simulink model "Tractive_System_model"  (R2025b)
settings: Solver=ode15s  StartTime=0  StopTime=85  MaxStep=1e-5  MinStep=1e-8  RelTol=1e-3  AbsTol=1e-6
undefined symbols (not defined in the file): FL, FR, RL, RR
libraries: batteryecm_lib x280, fl_lib x56, nesl_utility x37, ee_lib x9, sdl_lib x9, simulink x1, slpidlib x1, autolibshared x1, eePmsmFieldOrientedControl x1, eePmsmFwController x1
(part 1 of 23)
settings Model: PacingRate=0.002200  Creator=muizz  LastModifiedBy=muizz
settings SolverCC: AutoScaleAbsTol=off  InitialStep=1e-6  MaxConsecutiveMinStep=10000  ZeroCrossAlgorithm=Adaptive
settings DebuggingCC: AlgebraicLoopMsg=none  IgnoredZcDiagnostic=none

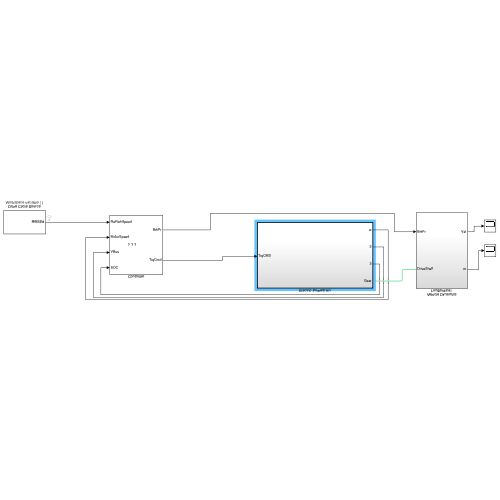
[thumbnail: Simulink's stored preview of the top-level diagram]
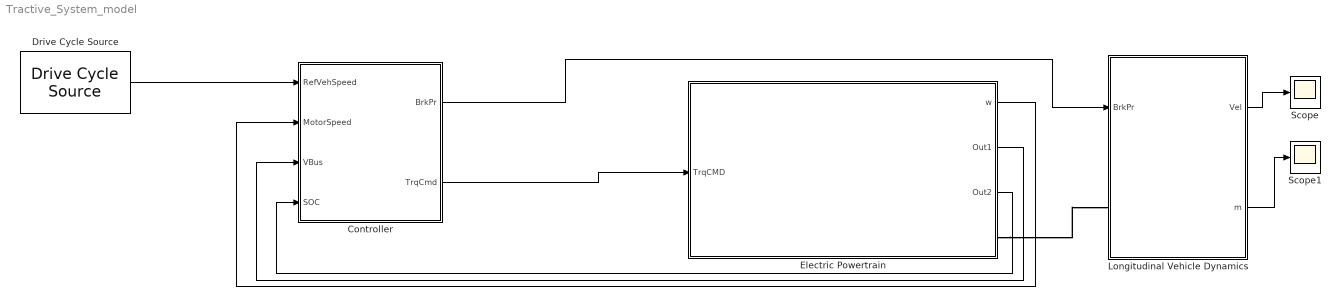
== system Tractive_System_model ==
  Controller : Subsystem
      mask Display: image('Images/brakeThrottle.png'); % Use "Edit Image" on toolstrip to change.
  Drive Cycle Source : autolibshared/Drive Cycle Source  cycleVar=Workspace variable  wsVar=fsdCycle  fileVar=cycleFTP75.mat  tfinal=""  cycleRepeat=on  outAccPort=off  outGearPort=off  gearList=No gear data  t_wot1=5  xdot_woto=0  xdot_wot1=30  t_wot2=20  xdot_wot2=0  t_wotend=30  srcUnit=m/s  outUnit=km/h  srcAccUnit=m/s/s  outAccUnit=m/s^2  dt=0  aMode=1  faultOption=off  velBnd=2  velBndUnit=mph  inUnit=m/s  timeBnd=1  failOption=off  stopSim=off  maxFaultCnt=10  maxFaultTime=2  maxTotFaultTime=15  traceOption=off  dtTrace=1  traceWindow=10  lastDCname=Custom Data Set  lastOutUnit=mph  lastDT=0  lastTB=1  lastSB=2  forceCalcBound=off
  Electric Powertrain : Subsystem  TreatAsAtomicUnit=on
  Longitudinal Vehicle Dynamics : Subsystem
  Scope : Scope
      settings: ActiveDisplayYMinimum=-1.2426886947971694  ActiveDisplayYMaximum=4.3208277664924974  DataLoggingVariableName=ScopeData5
  Scope1 : Scope
      settings: ActiveDisplayYMinimum=-1.4911055612240759E-16  ActiveDisplayYMaximum=1.5005598990985852E-16  DataLoggingVariableName=ScopeData6
  wires:
  Controller/2(TrqCmd) -> Electric Powertrain/1(TrqCMD)
  Electric Powertrain/1(w) -> Controller/2(MotorSpeed)
  Controller/1(BrkPr) -> Longitudinal Vehicle Dynamics/1(BrkPr)
  Drive Cycle Source/1 -> Controller/1(RefVehSpeed)
  Longitudinal Vehicle Dynamics/2(m) -> Scope1/1
  Longitudinal Vehicle Dynamics/1(Vel) -> Scope/1
  Electric Powertrain/2(Out1) -> Controller/3(VBus)
  Electric Powertrain/3(Out2) -> Controller/4(SOC)
  connections:
  Electric Powertrain/RConn1 -- Longitudinal Vehicle Dynamics/LConn1

== system Tractive_System_model/Controller ==
  RefVehSpeed : Inport
  MotorSpeed : Inport  Port=2
  VBus : Inport  Port=3
  SOC : Inport  Port=4
  Control : Subsystem
  Motor Speed Reference : Subsystem
  BrkPr : Outport
  TrqCmd : Outport  Port=2
  tag scope: Ref=global
  wires:
  RefVehSpeed/1 -> [Ref], Motor Speed Reference/1(VehSpd)
  MotorSpeed/1 -> Control/1(In1)
  Motor Speed Reference/1(MotorSpdRef) -> Control/2(Motor Speed Ref)  "Motor Speed Ref"
  VBus/1 -> Control/3(VBus)
  SOC/1 -> Control/4(SOC)
  Control/1(Pressure) -> BrkPr/1
  Control/2(MotCmdTrq) -> TrqCmd/1

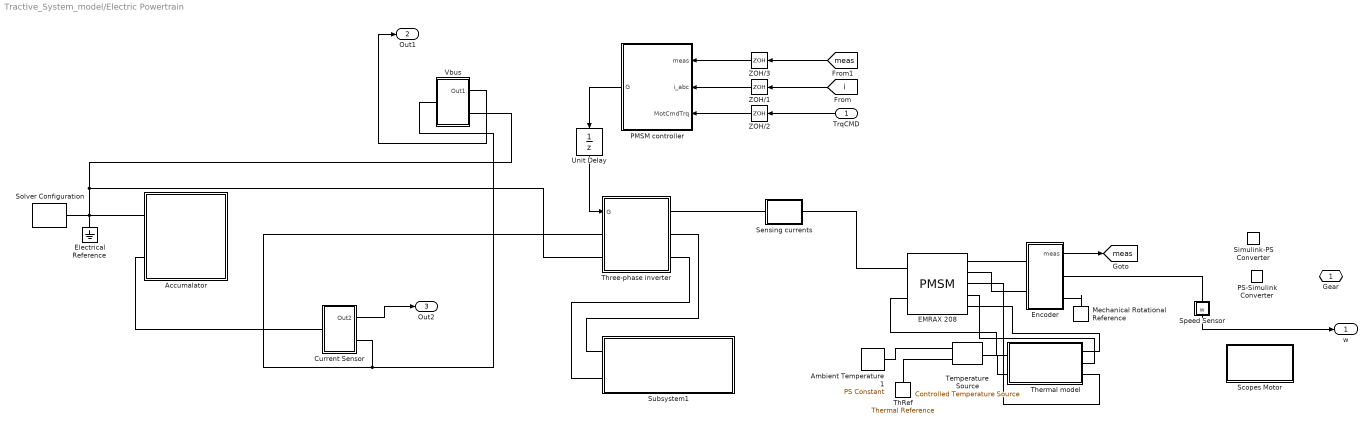
== system Tractive_System_model/Electric Powertrain ==
  TrqCMD : Inport
  Accumalator : Subsystem
  Ambient Temperature1 : fl_lib/Physical Signals/Sources/PS Constant  constant=300.15 K
  Current Sensor : Subsystem
  EMRAX 208 : ee_lib/Electromechanical/Permanent Magnet/PMSM  port_option=ee.enum.threePhasePort.composite  winding_type=ee.enum.electromech.statorconfiguration.wye  machine_param=ee.enum.pmsm.parameterization.constant  nPolePairs=10  pmflux_param=ee.enum.pmflux.fluxlinkage  pm_flux_linkage=0.23 Wb  torque_constant=0.916923438250803 % Datasheet derived N*m/A  back_emf_constant=0.916923438250803 % Datasheet derived V/(rad/s)  stator_param=ee.enum.statorparam.LdLqL0  Ld=0.138 mH  Lq=0.138 mH  idVec=[-200, 0, 200] A  iqVec=[-200, 0, 200] A  LdMatrix=0.0002 * ones(3, 3) H  LqMatrix=0.0002 * ones(3, 3) H  PmMatrix=0.1 * ones(3, 3) Wb  ktMatrix=0.18 * ones(3, 3) N*m/A  keMatrix=0.18 * ones(3, 3) V*s/rad  L0=0.00016 H  Ls=0.0002 H  Lm=-0.00002 H  Ms=0.00002 H  Rs=12 mOhm  zero_sequence=ee.enum.park.zerosequence.exclude  axes_param=ee.enum.rotorangle.daxis  loss_param=ee.enum.ironloss.none  losses_oc=[0, 0, 0] W  losses_sc=[0, 0, 0] W  f_losses=60 Hz  Isc_losses=95 A  J=256 kg*cm^2  lam=0 N*m*s/rad  i_d_specify=off  i_d_priority=None  i_d=0 A  i_d_nominal_specify=off  i_d_nominal_value=1  i_d_nominal_unit=A  i_q_specify=off  i_q_priority=None  i_q=0 A  i_q_nominal_specify=off  i_q_nominal_value=1  i_q_nominal_unit=A  torque_specify=off  torque_priority=High  torque=80 N*m  torque_nominal_specify=on  torque_nominal_value=80  torque_nominal_unit=N*m  angular_velocity_specify=off  angular_velocity_priority=High  angular_velocity=0 rpm  angular_velocity_nominal_specify=off  angular_velocity_nominal_value=1  angular_velocity_nominal_unit=rpm  angular_position_specify=off  angular_position_priority=High  angular_position=0 deg  angular_position_nominal_specify=off  angular_position_nominal_value=1  angular_position_nominal_unit=deg  alpha=3.93e-3 1/K  alpha_flux=-0.001 1/K  Tmeas=298.15 K  stator_thermal_mass=423.5 J/K  rotor_thermal_mass=2714 J/K  Rm_percent_rotor=90  Rd_percent_rotor=30  temperatureA_specify=off  temperatureA_priority=High  temperatureA=25 degC  temperatureA_nominal_specify=off  temperatureA_nominal_value=1  temperatureA_nominal_unit=degC  temperatureB_specify=off  temperatureB_priority=High  temperatureB=25 degC  temperatureB_nominal_specify=off  temperatureB_nominal_value=1  temperatureB_nominal_unit=degC  temperatureC_specify=off  temperatureC_priority=High  temperatureC=25 degC  temperatureC_nominal_specify=off  temperatureC_nominal_value=1  temperatureC_nominal_unit=degC  temperatureR_specify=off  temperatureR_priority=High  temperatureR=25 degC  temperatureR_nominal_specify=off  temperatureR_nominal_value=1  temperatureR_nominal_unit=degC
      settings: InternalSimscapePortConfiguration="{\"Bottom\":[],\"Left\":[{\"id\":\"N\",\"label\":\"~\",\"type\":\"foundation.electrical.three_phase\"},{\"id\":\"HR\",\"label\":\"HR\",\"type\":\"foundation.thermal.thermal\"}],\"Right\":[{\"id\":\"R\",\"label\":\"R\",\"type\":\"foundation.mechanical.rotational.rotational\"},{\"id\":\"C\",\"label\":\"C\",\"type\":\"foundation.mechanical.rotational.rotational\"},{\"id\":\"HA\",\"label\":\"HA\",\"type\":\"foundation.thermal.thermal\"},{\"id\":\"HB\",\"label\":\"HB\",\"type\":\"foundation.thermal.thermal\"},{\"id\":\"HC\",\"label\":\"HC\",\"type\":\"foundation.thermal.thermal\"}],\"Top\":[]}"
  Electrical Reference : fl_lib/Electrical/Electrical Elements/Electrical Reference
  Encoder : Subsystem
  Mechanical Rotational Reference : fl_lib/Mechanical/Rotational Elements/Mechanical Rotational Reference
  PMSM controller : Subsystem
  PS-Simulink Converter : nesl_utility/PS-Simulink Converter  PhysicalDomain=network_engine_domain  SubClassName=ps_output  LeftPortType=input  RightPortType=output  PseudoPeriodic=off  Frequencies=[]  VectorFormat=inherit  Unit=inherit  AffineConversion=off
  Scopes Motor : Subsystem
  Sensing currents : Subsystem
      mask Display: disp('i')
  Simulink-PS Converter : nesl_utility/Simulink-PS Converter  PhysicalDomain=network_engine_domain  SubClassName=ps_input  LeftPortType=input  RightPortType=output  PseudoPeriodic=off  Frequencies=[]  NoiseDistribution=none  NoiseParameters=[]  Unit=1  AffineConversion=off  FilteringAndDerivatives=provide  SimscapeFilterOrder=1  InputFilterTimeConstant=0.001  UdotUserProvided=0
  Solver Configuration : nesl_utility/Solver Configuration  PhysicalDomain=network_engine_domain  SubClassName=solver  LeftPortType=input  RightPortType=generic  Tones=[]  Harmonics=[]  SimulateNoise=off  Profile=off  UseLocalSampling=off  EnableSwitchedLinearOptims=on  FrequencyDomain=off  UseCCode=off  RelTol=0.001  AbsTol=0.001  MinStep=1e-09  ToWorkspace=off  RevertToSquareIcSolve=off  NumHomotopyIterations=100  PhasorMode=off  PhasorModeNumHarmonics=1  ConsistencySolver=NEWTON_XTOL_AFTER_FTOL  IndexReductionMethod=DerivativeReplacement  DoDC=off  ResidualTolerance=1e-09  ConsistencyTolSource=GLOBAL  ConsistencyAbsTol=0.001  ConsistencyRelTol=0.001  ConsistencyTolFactor=1e-4  UseLocalSolver=off  LocalSolverChoice=NE_BACKWARD_EULER_ADVANCER  ResolveIndetEquations=on  FunctionEvalNumThread=1  LocalSolverSampleTime=1e-04  DoFixedCost=off  MaxNonlinIter=3  MaxModeIter=2  ComputeImpulses=off  ImpulseIterations=2  LinearAlgebra=auto  LinearAlgebraNumThread=0  EquationFormulation=NE_TIME_EF  DelaysMemoryBudget=1024  AutomaticFiltering=on  FilteringTimeConstant=0.001  PartitionStorageMethod=AS_NEEDED  PartitionMemoryBudget=1024  PartitionMethod=ROBUST  MultibodyUseLocalSolver=off  MultibodyLocalSolverChoice=ODE1  MultibodyLocalSolverSampleTime=0.005
  Speed Sensor : Subsystem
      mask Display: disp('w')
  Subsystem1 : Subsystem
  Temperature Source : fl_lib/Thermal/Thermal Sources/Controlled Temperature Source
  ThRef : fl_lib/Thermal/Thermal Elements/Thermal Reference
  Thermal model : Subsystem  Tag=PublishSubsystem
  Three-phase inverter : Subsystem
  Unit Delay : UnitDelay  SampleTime=-1  HasFrameUpgradeWarning=on
  Vbus : Subsystem
  ZOH/1 : ZeroOrderHold  SampleTime=2e-05
  ZOH/2 : ZeroOrderHold  SampleTime=2e-05
  ZOH/3 : ZeroOrderHold  SampleTime=2e-05
  Gear : PMIOPort  Side=Right
  w : Outport
  Out1 : Outport  Port=2
  Out2 : Outport  Port=3
  tag scope: meas=global
  wires:
  Unit Delay/1 -> Three-phase inverter/1(G)
  [meas] -> ZOH/3/1
  PMSM controller/1(G) -> Unit Delay/1
  Speed Sensor/1(w) -> w/1
  Encoder/1(meas) -> [meas]
  [i] -> ZOH/1/1
  ZOH/2/1 -> PMSM controller/3(MotCmdTrq)
  ZOH/1/1 -> PMSM controller/2(i_abc)
  ZOH/3/1 -> PMSM controller/1(meas)
  TrqCMD/1 -> ZOH/2/1
  Current Sensor/1(Out2) -> Out2/1
  Vbus/1(Out1) -> Out1/1
  connections:
  EMRAX 208/RConn2 -- Encoder/LConn2
  Thermal model/RConn1 -- EMRAX 208/RConn5
  Temperature Source/LConn1 -- Thermal model/LConn2
  Sensing currents/LConn1 -- Three-phase inverter/RConn1
  ThRef/LConn1 -- Temperature Source/RConn2
  Temperature Source/RConn1 -- Ambient Temperature1/RConn1
  EMRAX 208/RConn4 -- Thermal model/RConn2
  Speed Sensor/LConn1 -- Encoder/RConn1
  Sensing currents/RConn1 -- EMRAX 208/LConn1
  Three-phase inverter/LConn2 -- Vbus/RConn1 -- Solver Configuration/RConn1 -- Electrical Reference/LConn1 -- Accumalator/LConn1
  Thermal model/RConn3 -- EMRAX 208/RConn3
  EMRAX 208/RConn1 -- Encoder/LConn1
  Mechanical Rotational Reference/LConn1 -- Encoder/RConn2
  Thermal model/LConn1 -- EMRAX 208/LConn2
  Three-phase inverter/RConn2 -- Subsystem1/LConn1
  Three-phase inverter/RConn3 -- Subsystem1/LConn2
  Current Sensor/LConn1 -- Accumalator/LConn2
  Current Sensor/RConn1 -- Vbus/LConn1 -- Three-phase inverter/LConn1

== system Tractive_System_model/Longitudinal Vehicle Dynamics ==
  BrkPr : Inport
  Brakes : Subsystem
  Bus Selector2 : BusSelector  OutputSignals=RoadGrade,Wind
  Chassis and Tires : Subsystem
  Env : Subsystem
  PS Gain1 : fl_lib/Physical Signals/Functions/PS Gain  gain=1
  Sensor Subsystem : Subsystem
  Simulink-PS Converter : nesl_utility/Simulink-PS Converter  PhysicalDomain=network_engine_domain  SubClassName=ps_input  LeftPortType=input  RightPortType=output  PseudoPeriodic=off  Frequencies=[]  NoiseDistribution=none  NoiseParameters=[]  Unit=1  AffineConversion=off  FilteringAndDerivatives=provide  SimscapeFilterOrder=1  InputFilterTimeConstant=0.001  UdotUserProvided=0
  Simulink-PS Converter2 : nesl_utility/Simulink-PS Converter  PhysicalDomain=network_engine_domain  SubClassName=ps_input  LeftPortType=input  RightPortType=output  PseudoPeriodic=off  Frequencies=[]  NoiseDistribution=none  NoiseParameters=[]  Unit=rad  AffineConversion=off  FilteringAndDerivatives=provide  SimscapeFilterOrder=1  InputFilterTimeConstant=0.001  UdotUserProvided=0
  Simulink-PS Converter3 : nesl_utility/Simulink-PS Converter  PhysicalDomain=network_engine_domain  SubClassName=ps_input  LeftPortType=input  RightPortType=output  PseudoPeriodic=off  Frequencies=[]  NoiseDistribution=none  NoiseParameters=[]  Unit=N/m^2  AffineConversion=off  FilteringAndDerivatives=provide  SimscapeFilterOrder=1  InputFilterTimeConstant=0.001  UdotUserProvided=0
  Simulink-PS Converter4 : nesl_utility/Simulink-PS Converter  PhysicalDomain=network_engine_domain  SubClassName=ps_input  LeftPortType=input  RightPortType=output  PseudoPeriodic=off  Frequencies=[]  NoiseDistribution=none  NoiseParameters=[]  Unit=m/s  AffineConversion=off  FilteringAndDerivatives=provide  SimscapeFilterOrder=1  InputFilterTimeConstant=0.001  UdotUserProvided=0
  DriveShaft : PMIOPort  Side=Left
  Vel : Outport
  Out Bus Element : Outport  Port=2  PortName=m  Element=Brakes
  Out Bus Element1 : Outport  Port=2  PortName=m  Element=Chassis
  wires:
  BrkPr/1 -> Simulink-PS Converter3/1
  Env/1(Env) -> Bus Selector2/1
  Brakes/1(m) -> Out Bus Element/1
  Bus Selector2/2 -> Simulink-PS Converter4/1  "<Wind>"
  Bus Selector2/1 -> Simulink-PS Converter2/1  "<RoadGrade>"
  Chassis and Tires/1(m) -> Out Bus Element1/1
  Sensor Subsystem/1(kph) -> Vel/1, Env/1(m)
  connections:
  PS Gain1/LConn1 -- Brakes/LConn1 -- Simulink-PS Converter3/RConn1
  Chassis and Tires/RConn2 -- Simulink-PS Converter4/RConn1
  PS Gain1/RConn1 -- Brakes/LConn2
  Chassis and Tires/LConn2 -- DriveShaft/RConn1
  Chassis and Tires/LConn1 -- Brakes/RConn1
  Chassis and Tires/RConn1 -- Simulink-PS Converter2/RConn1
  Chassis and Tires/RConn3 -- Sensor Subsystem/LConn1

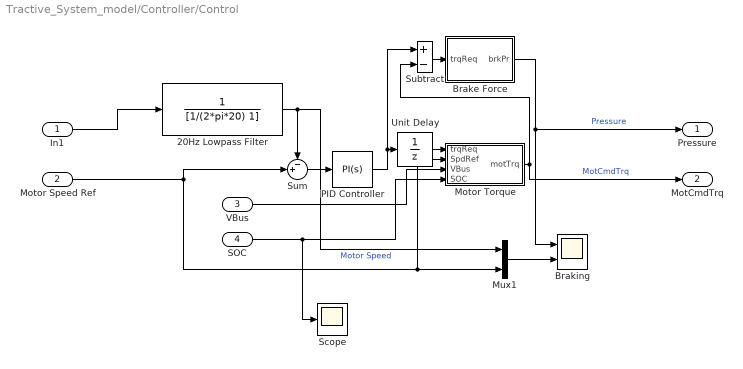
== system Tractive_System_model/Controller/Control ==
  In1 : Inport
  Motor Speed Ref : Inport  Port=2
  VBus : Inport  Port=3
  SOC : Inport  Port=4
  20Hz Lowpass Filter : TransferFcn  Denominator=[1/(2*pi*20) 1]
  Brake Force : Subsystem
  Braking : Scope  NumInputPorts=2
      settings: ActiveDisplayYMinimum=-6.26637814618E+6  ActiveDisplayYMaximum=5.639740331562E+7
  Motor Torque : Subsystem
  Mux1 : Mux  Inputs=2
  PID Controller : slpidlib/PID Controller  Controller=PI  Form=Parallel  TimeDomain=Continuous-time  UseExternalTs=off  SampleTime=-1  IntegratorMethod=Forward Euler  FilterMethod=Forward Euler  ControllerParametersSource=internal  P=0.5  I=1e-03  UseKiTs=off  D=0  UseExternalDerivativeSource=off  N=100  UseFilter=on  TunerSelectOption=Transfer Function Based (PID Tuner App)  InitialConditionSource=internal  InitialConditionForIntegrator=0  InitialConditionForFilter=0  DifferentiatorICPrevScaledInput=0  ExternalReset=none  TrackingMode=off  Kt=1  LimitOutput=off  SatLimitsSource=internal  UpperSaturationLimit=inf  LowerSaturationLimit=-inf  LinearizeAsGain=on  AntiWindupMode=none  Kb=1  LimitIntegrator=off  UpperIntegratorSaturationLimit=inf  LowerIntegratorSaturationLimit=-inf  POutMin=[]  POutMax=[]  IOutMin=[]  IOutMax=[]  DOutMin=[]  DOutMax=[]  NOutMin=[]  NOutMax=[]  SumOutMin=[]  SumOutMax=[]  SaturationOutMin=[]  SaturationOutMax=[]  PParamMin=[]  PParamMax=[]  IParamMin=[]  IParamMax=[]  DParamMin=[]  DParamMax=[]  NParamMin=[]  NParamMax=[]  KbParamMin=[]  KbParamMax=[]  KtParamMin=[]  KtParamMax=[]  KbOutMin=[]  KbOutMax=[]  KtOutMin=[]  KtOutMax=[]  IntegratorOutMin=[]  IntegratorOutMax=[]  FilterOutMin=[]  FilterOutMax=[]  SumI1OutMin=[]  SumI1OutMax=[]  SumI2OutMin=[]  SumI2OutMax=[]  SumI3OutMin=[]  SumI3OutMax=[]  SumI4OutMin=[]  SumI4OutMax=[]  SumDOutMin=[]  SumDOutMax=[]  DifferentiatorOutMin=[]  DifferentiatorOutMax=[]  FilterDiffOutCoefMin=[]  FilterDiffOutCoefMax=[]  ReciprocalOutMin=[]  ReciprocalOutMax=[]  SumDenOutMin=[]  SumDenOutMax=[]  SumNumOutMin=[]  SumNumOutMax=[]  DivideOutMin=[]  DivideOutMax=[]  UdiffTsProdOutMin=[]  UdiffTsProdOutMax=[]  NTsProdOutMin=[]  NTsProdOutMax=[]  UintegralTsProdOutMin=[]  UintegralTsProdOutMax=[]  UngainTsProdOutMin=[]  UngainTsProdOutMax=[]  ClampingZeroOutDataTypeStr=Inherit: Inherit via back propagation  ClampingZeroOutMin=[]  ClampingZeroOutMax=[]  FilterDenConstantOutDataTypeStr=Inherit: Inherit via back propagation  FilterDenConstantOutMin=[]  FilterDenConstantOutMax=[]  PCopyOutDataTypeStr=Inherit: Inherit via back propagation  PCopyOutMin=[]  PCopyOutMax=[]  NCopyOutDataTypeStr=Inherit: Inherit via back propagation  NCopyOutMin=[]  NCopyOutMax=[]  IntegratorContinuousStateAttributes=''  IntegratorStateMustResolveToSignalObject=off  IntegratorRTWStateStorageClass=Auto  FilterContinuousStateAttributes=''  FilterStateMustResolveToSignalObject=off  FilterRTWStateStorageClass=Auto  ParallelPVariant=InternalParameters  IdealPVariant=Disabled  IVariant=InternalParameters  DVariant=Disabled  IntegratorVariant=Continuous  SatVariant=Disabled  AWVariant=Passthrough  PCopyVariant=Disabled  TRVariant=Disabled  FdbkBlocksVariant=Forward  IdealPFdbkVariant=Disabled  SatFdbkVariant=Disabled  DerivativeFilterVariant=Disabled  NVariant=Disabled  NCopyVariant=Disabled_SignalSpec  FilterICVariant=Disabled  IntegratorICVariant=InternalICs  ExternalResetVariant=Disabled  TRSumVariant=Passthrough  SumFdbkVariant=Disabled  SumVariant=Sum_PI  TsampFilterVariant=InternalTs  TsampNgainVariant=Passthrough  TsampIntegralVariant=Disabled_SignalSpec  ExternalSaturationOutDataTypeStr=Inherit: Same as second input  DerivativeSourceVariant=Disabled  PreIntVariant=InternalPreInt
  Scope : Scope
      settings: DataLoggingVariableName=ScopeData7
  Subtract : Sum  Inputs=+-
  Sum : Sum  Inputs=-+|
  Unit Delay : UnitDelay  SampleTime=-1  HasFrameUpgradeWarning=on
  Pressure : Outport
  MotCmdTrq : Outport  Port=2
  wires:
  Sum/1 -> PID Controller/1
  Motor Torque/1(motTrq) -> MotCmdTrq/1, Subtract/2  "MotCmdTrq"
  20Hz Lowpass Filter/1 -> Sum/1, Mux1/1  "Motor Speed"
  Brake Force/1(brkPr) -> Pressure/1, Braking/1  "Pressure"
  Mux1/1 -> Braking/2
  Subtract/1 -> Brake Force/1(trqReq)
  Motor Speed Ref/1 -> Motor Torque/2(SpdRef), Mux1/2, Sum/2
  VBus/1 -> Motor Torque/3(VBus)
  SOC/1 -> Scope/1, Motor Torque/4(SOC)
  In1/1 -> 20Hz Lowpass Filter/1
  PID Controller/1 -> Subtract/1, Unit Delay/1
  Unit Delay/1 -> Motor Torque/1(trqReq)

== system Tractive_System_model/Controller/Motor Speed Reference ==
  note: Motor Reducer Output Shaft to Wheels
  VehSpd : Inport  Unit=km/hr
  Constant1 : Constant  Value=20.32
  Differential : Constant  Value=4.28
  Divide : Product  Inputs=*/
  Gain : Gain  Gain=2*pi
  Gain1 : Gain  Gain=1/100
  Product : Product
  Signal Specification : SignalSpecification  Unit=m/min
  Unit Conversion : UnitConversion
  MotorSpdRef : Outport  Unit=rpm  VectorParamsAs1DForOutWhenUnconnected=off
  wires:
  VehSpd/1 -> Unit Conversion/1
  Unit Conversion/1 -> Signal Specification/1
  Signal Specification/1 -> Divide/1
  Constant1/1 -> Gain1/1  "cm"
  Gain/1 -> Divide/2  "2*pi*R (m)"
  Divide/1 -> Product/1  "tireRpmRef"
  Product/1 -> MotorSpdRef/1  "motorRpmRef"
  Gain1/1 -> Gain/1  "m"
  Differential/1 -> Product/2

== system Tractive_System_model/Electric Powertrain/Accumalator ==
  Module  four : Subsystem
  Module Five1 : Subsystem
  Module One1 : Subsystem
  Module Three1 : Subsystem
  "Module Two " : Subsystem
  - : PMIOPort  Side=Left
  + : PMIOPort  Port=2  Side=Left
  connections:
  "Module Two "/LConn2 -- Module Three1/LConn1
  Module Three1/LConn2 -- Module  four/LConn1
  Module One1/LConn2 -- "Module Two "/LConn1
  Module  four/LConn2 -- Module Five1/LConn1
  Module Five1/LConn2 -- -/RConn1
  Module One1/LConn1 -- +/RConn1

== system Tractive_System_model/Electric Powertrain/Current Sensor ==
  Current Sensor : fl_lib/Electrical/Electrical Sensors/Current Sensor
  Current sensing : nesl_utility/PS-Simulink Converter  PhysicalDomain=network_engine_domain  SubClassName=ps_output  LeftPortType=input  RightPortType=output  PseudoPeriodic=off  Frequencies=[]  VectorFormat=inherit  Unit=inherit  AffineConversion=off
  Integrator : Integrator  InitialCondition=1
  Saturation : Saturate  UpperLimit=1  LowerLimit=0
  Scope1 : Scope
      settings: ActiveDisplayYMinimum=-20.563211553740629  ActiveDisplayYMaximum=64.19065525989943  DataLoggingVariableName=ScopeData4
  Conn1 : PMIOPort  Side=Left
  Conn2 : PMIOPort  Port=2  Side=Right
  Out2 : Outport
  wires:
  Saturation/1 -> Out2/1
  Current sensing/1 -> Integrator/1, Scope1/1
  Integrator/1 -> Saturation/1
  connections:
  Current Sensor/LConn1 -- Conn1/RConn1
  Current Sensor/RConn2 -- Conn2/RConn1
  Current Sensor/RConn1 -- Current sensing/LConn1

== system Tractive_System_model/Electric Powertrain/Encoder ==
  Ideal Rotational Motion Sensor : fl_lib/Mechanical/Mechanical Sensors/Ideal Rotational Motion Sensor  reference=foundation.enum.MeasurementReference.difference  acceleration_port=false  velocity_port=true  position_port=true  wrap_angle=simscape.enum.onoff.off  offset=0 deg
  Ideal Torque Sensor : fl_lib/Mechanical/Mechanical Sensors/Ideal Torque Sensor
  Mux : Mux  Inputs=2
  PS-Simulink Converter : nesl_utility/PS-Simulink Converter  PhysicalDomain=network_engine_domain  SubClassName=ps_output  LeftPortType=input  RightPortType=output  PseudoPeriodic=off  Frequencies=[]  VectorFormat=1-D array  Unit=rad/s  AffineConversion=off
  PS-Simulink Converter1 : nesl_utility/PS-Simulink Converter  PhysicalDomain=network_engine_domain  SubClassName=ps_output  LeftPortType=input  RightPortType=output  PseudoPeriodic=off  Frequencies=[]  VectorFormat=1-D array  Unit=rad  AffineConversion=off
  PS-Simulink Converter2 : nesl_utility/PS-Simulink Converter  PhysicalDomain=network_engine_domain  SubClassName=ps_output  LeftPortType=input  RightPortType=output  PseudoPeriodic=off  Frequencies=[]  VectorFormat=1-D array  Unit=N*m  AffineConversion=off
  1L : PMIOPort  Side=Left
  2L : PMIOPort  Port=2  Side=Left
  1R : PMIOPort  Port=3  Side=Right
  2R : PMIOPort  Port=4  Side=Right
  meas : Outport  VectorParamsAs1DForOutWhenUnconnected=off
  tag scope: trqMotor=global, wMotor=global
  wires:
  PS-Simulink Converter2/1 -> [trqMotor]
  Mux/1 -> meas/1
  PS-Simulink Converter1/1 -> Mux/2
  PS-Simulink Converter/1 -> [wMotor], Mux/1
  connections:
  Ideal Torque Sensor/RConn2 -- PS-Simulink Converter2/LConn1
  1L/RConn1 -- Ideal Torque Sensor/LConn1
  2R/RConn1 -- 2L/RConn1 -- Ideal Rotational Motion Sensor/RConn1
  Ideal Rotational Motion Sensor/LConn1 -- 1R/RConn1 -- Ideal Torque Sensor/RConn1
  Ideal Rotational Motion Sensor/RConn2 -- PS-Simulink Converter/LConn1
  Ideal Rotational Motion Sensor/RConn3 -- PS-Simulink Converter1/LConn1

== system Tractive_System_model/Electric Powertrain/PMSM controller ==
  meas : Inport
  i_abc : Inport  Port=2
  MotCmdTrq : Inport  Port=3
  Bus Selector : BusSelector  OutputSignals=iabc [A],Reference,TqRef [N*m],idq [A]
  Demux1 : Demux  Outputs=2
  PMSM Field-Oriented Control : eePmsmFieldOrientedControl/PMSM Field-Oriented Control  winding_type=Wye-wound  CtrlMode=Torque control  Vnom=572  Pmax=80000  Tmax=150  p=10  Vdc_on=30  Ts=1e-5  Tsc=1e-5  CtrlType=PI control  Kp_w=60  Ki_w=300*2  Kv_w=1  Kaw_w=1000  RefType=Zero d-axis control  rpmVec=[0, 3000]  TqVec=[-100, 0, 100]  VdcVec=[300, 350]  PWMMode=SPWM: sinusoidal PWM  ModFactor=1  idMatrix=zeros(2,3,2)  iqMatrix=zeros(2,3,2)  psim=0.0275  Ld=0.00024  Lq=0.00029  Rs=0.01  AxisAlignment=Q-axis  Kp_id=0.540  Ki_id=5.7  Kaw_id=1000  Kp_iq=0.540  Ki_iq=5.7  Kaw_iq=1000  AxisPrio=Q-axis  ActZC=off  ActFF=on  ParamTypeFF=Constant parameters  LdFF=0.0002  LqFF=0.0002  psimFF=0.0275  idVect=[-200, 0, 200]  iqVect=[-200, 0, 200]  LdMatrix=0.0002 * ones(3, 3)  LqMatrix=0.0002 * ones(3, 3)  psimMatrix=0.04 * ones(3, 3)  CPWMMode=SPWM: sinusoidal PWM  fsw=10000
  PMSM Field-Weakening Controller : eePmsmFwController/PMSM Field-Weakening Controller  Commented=on  Mth=1  Kfw=100  Kaw=10  Ts=-1
      settings: LibrarySourceBlock=|
      | ee_sl_lib/PMSM Control/PMSM Field-Weakening
      | Controller
  Vdc : Constant  Value=572  SampleTime=2e-05
  G : Outport  VectorParamsAs1DForOutWhenUnconnected=off
  tag scope: G=global, iMotor=global, idq=global, trqDemand=global, wDemand=global
  wires:
  PMSM Field-Oriented Control/1 -> G/1, [G]
  Vdc/1 -> PMSM Field-Oriented Control/5
  PMSM Field-Oriented Control/2 -> Bus Selector/1
  i_abc/1 -> PMSM Field-Oriented Control/2
  meas/1 -> Demux1/1
  Demux1/1 -> PMSM Field-Oriented Control/3
  Demux1/2 -> PMSM Field-Oriented Control/4
  Bus Selector/1 -> [iMotor]  "<iabc [A]>"
  Bus Selector/2 -> [wDemand]  "<Reference>"
  Bus Selector/3 -> [trqDemand]  "<TqRef [N*m]>"
  Bus Selector/4 -> [idq]  "<idq [A]>"
  MotCmdTrq/1 -> PMSM Field-Oriented Control/1

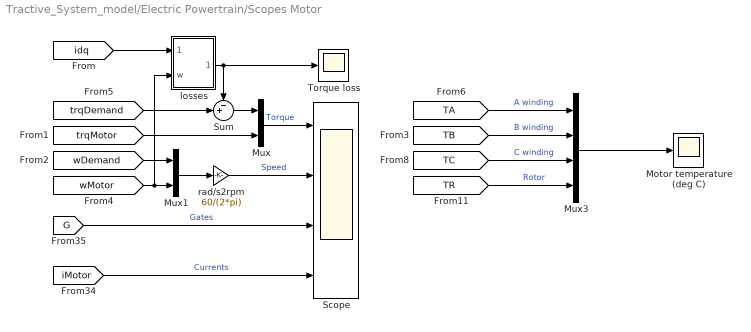
== system Tractive_System_model/Electric Powertrain/Scopes Motor ==
  Motor temperature (deg C) : Scope
      settings: Title=Motor temperature (deg C)  ActiveDisplayYMinimum=13.563074138954487  ActiveDisplayYMaximum=33.98024222270584  DataLoggingMaxPoints=500000  DataLoggingDecimation=10
  Mux : Mux  Inputs=2
  Mux1 : Mux  Inputs=2
  Mux3 : Mux
  Scope : Scope  NumInputPorts=4
      settings: Title=Demanded and achieved torques  ActiveDisplayYMinimum=-8.8227194148565182  ActiveDisplayYMaximum=43.531185116331216
  Sum : Sum  Inputs=-+|
  Torque loss : Scope
      settings: ActiveDisplayYMinimum=-15.776290162311993  ActiveDisplayYMaximum=9.8949447297595938
  losses : Subsystem
  rad/s2rpm : Gain  Gain=60/(2*pi)
  wires:
  [TC] -> Mux3/3  "C winding"
  [TR] -> Mux3/4  "Rotor"
  [TB] -> Mux3/2  "B winding"
  [TA] -> Mux3/1  "A winding"
  Mux3/1 -> Motor temperature (deg C)/1
  rad/s2rpm/1 -> Scope/2  "Speed"
  [G] -> Scope/3  "Gates"
  [wDemand] -> Mux1/1
  [wMotor] -> losses/2(w), Mux1/2
  [iMotor] -> Scope/4  "Currents"
  [trqMotor] -> Mux/2
  Mux1/1 -> rad/s2rpm/1
  Mux/1 -> Scope/1  "Torque"
  [idq] -> losses/1(idq)
  losses/1(tq_loss) -> Torque loss/1, Sum/1
  Sum/1 -> Mux/1
  [trqDemand] -> Sum/2

== system Tractive_System_model/Electric Powertrain/Sensing currents ==
  Current Sensor : ee_lib/Sensors & Transducers/Current Sensor (Three-Phase)
  PS-Simulink Converter : nesl_utility/PS-Simulink Converter  PhysicalDomain=network_engine_domain  SubClassName=ps_output  LeftPortType=input  RightPortType=output  PseudoPeriodic=off  Frequencies=[]  VectorFormat=1-D array  Unit=A  AffineConversion=off
  Conn1 : PMIOPort  Side=Left
  Conn2 : PMIOPort  Port=2  Side=Right
  tag scope: i=global
  wires:
  PS-Simulink Converter/1 -> [i]
  connections:
  Current Sensor/RConn1 -- PS-Simulink Converter/LConn1
  Conn2/RConn1 -- Current Sensor/RConn2
  Conn1/RConn1 -- Current Sensor/LConn1

== system Tractive_System_model/Electric Powertrain/Speed Sensor ==
  Mechanical Rotational Reference1 : fl_lib/Mechanical/Rotational Elements/Mechanical Rotational Reference
  Motion Sensor : fl_lib/Mechanical/Mechanical Sensors/Ideal Rotational Motion Sensor  reference=foundation.enum.MeasurementReference.difference  acceleration_port=false  velocity_port=true  position_port=true  wrap_angle=simscape.enum.onoff.off  offset=0 rad
  PS Terminator : fl_lib/Physical Signals/Sinks/PS Terminator
  PS-Simulink Converter 2 : nesl_utility/PS-Simulink Converter  PhysicalDomain=network_engine_domain  SubClassName=ps_output  LeftPortType=input  RightPortType=output  PseudoPeriodic=off  Frequencies=[]  VectorFormat=1-D array  Unit=rpm  AffineConversion=off
  R : PMIOPort  Side=Left
  w : Outport
  wires:
  PS-Simulink Converter 2/1 -> w/1
  connections:
  Motion Sensor/RConn2 -- PS-Simulink Converter 2/LConn1
  Motion Sensor/RConn1 -- Mechanical Rotational Reference1/LConn1
  Motion Sensor/RConn3 -- PS Terminator/LConn1
  Motion Sensor/LConn1 -- R/RConn1

== system Tractive_System_model/Electric Powertrain/Subsystem1 ==
  Inverter Power_loss : Scope
      settings: ActiveDisplayYMinimum=494.35276847042581  ActiveDisplayYMaximum=494.59601568207728  DataLoggingVariableName=ScopeData3
  PS Lookup Table (2D) : fl_lib/Physical Signals/Lookup Tables/PS Lookup Table (2D)  x1=[100, 150, 200, 250, 300, 350, 400, 450, 500, 550, 600, 650, 700, 750, 800] V  x2=[100, 150, 200, 250, 300, 350, 400, 450, 500, 550, 600] A  f=|  interp_method=simscape.enum.interpolation.smooth  extrap_method=simscape.enum.extrapolation.nearest
      | [199.5, 318, 436.5, 580.5, 724.5, 899.8, 1075, 1267.5, 1460, 1692.5, 1925;
      | 230.3, 362.3, 494.3, 651.8, 809.3, 998.4, 1187.5, 1393.8, 1600, 1843.8, 2087.5;
      | 261, 406.5, 552, 723, 894, 1097, 1300, 1520, 1740, 1995, 2250;
      | 291.8, 450.8, 609.8, 794.3, 978.8, 1195.6, 1412.5, 1646.3, 1880, 2146.3, 2412.5;
      | 322.5, 495, 667.5, 865.5, 1063.5, 1294.3, 1525, 1772.5, 2020, 2297.5, 2575;
      | 353.3, 539.3, 725.3, 936.8, 1148.3, 1392.9, 1637.5, 1898.8, 2160, 2448.8, 2737.5;
      | 384, 583.5, 783, 1008, 1233, 1491.5, 1750, 2025, 2300, 2600, 2900;
      | 416.3, 629.3, 842.3, 1081.5, 1320.8, 1591.6, 1862.5, 2156.3, 2450, 2768.8, 3087.5;
      | 448.5, 675, 901.5, 1155, 1408.5, 1691.8, 1975, 2287.5, 2600, 2937.5, 3275;
      | 480.8, 720.8, 960.8, 1228.5, 1496.3, 1791.9, 2087.5, 2418.8, 2750, 3106.3, 3462.5;
      | 513, 766.5, 1020, 1302, 1584, 1892, 2200, 2550, 2900, 3275, 3650;
      | 545.3, 812.6, 1080, 1378.5, 1677, 2006, 2335, 2698.8, 3062.5, 3462.5, 3862.5;
      | 577.5, 858.8, 1140, 1455, 1770, 2120, 2470, 2847.5, 3225, 3650, 4075;
      | 609.8, 904.9, 1200, 1531.5, 1863, 2234, 2605, 2996.3, 3387.5, 3837.5, 4287.5;
      | 642, 951, 1260, 1608, 1956, 2348, 2740, 3145, 3550, 4025, 4500] W
  PS-Simulink Converter : nesl_utility/PS-Simulink Converter  PhysicalDomain=network_engine_domain  SubClassName=ps_output  LeftPortType=input  RightPortType=output  PseudoPeriodic=off  Frequencies=[]  VectorFormat=inherit  Unit=W  AffineConversion=off
  ARMS_IN : PMIOPort  Side=Left
  VDC_IN : PMIOPort  Port=2  Side=Left
  wires:
  PS-Simulink Converter/1 -> Inverter Power_loss/1
  connections:
  ARMS_IN/RConn1 -- PS Lookup Table (2D)/LConn2
  VDC_IN/RConn1 -- PS Lookup Table (2D)/LConn1
  PS-Simulink Converter/LConn1 -- PS Lookup Table (2D)/RConn1

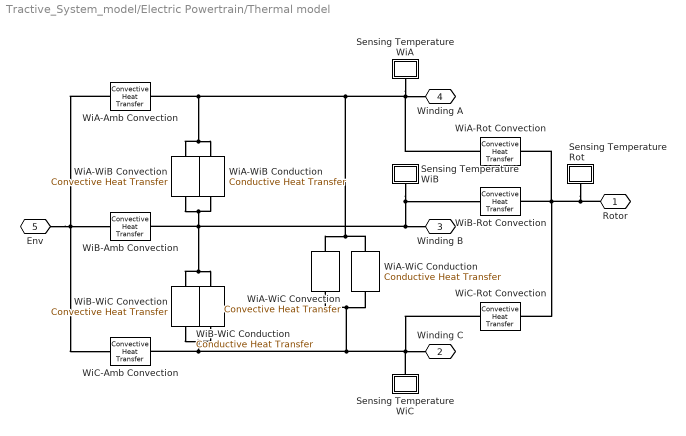
== system Tractive_System_model/Electric Powertrain/Thermal model ==
  Sensing Temperature Rot : Subsystem
      mask Display: disp('TR')
  Sensing Temperature WiA : Subsystem
      mask Display: disp('TA')
  Sensing Temperature WiB : Subsystem
      mask Display: disp('TB')
  Sensing Temperature WiC : Subsystem
      mask Display: disp('TC')
  WiA-Amb Convection : fl_lib/Thermal/Thermal Elements/Convective Heat Transfer  thermal_type=foundation.enum.constant_variable.constant  area=0.1 m^2  heat_tr_coeff=20 W/(m^2 * K)  min_heat_tr_coeff=1e-3 W/(K*m^2)  T_specify=off  T_priority=None  T=0 K  T_nominal_specify=off  T_nominal_value=1  T_nominal_unit=K  Q_specify=off  Q_priority=None  Q=0 J/s  Q_nominal_specify=off  Q_nominal_value=1  Q_nominal_unit=J/s
  WiA-Rot Convection : fl_lib/Thermal/Thermal Elements/Convective Heat Transfer  thermal_type=foundation.enum.constant_variable.constant  area=0.02 m^2  heat_tr_coeff=200 W/(m^2 * K)  min_heat_tr_coeff=1e-3 W/(K*m^2)  T_specify=off  T_priority=None  T=0 K  T_nominal_specify=off  T_nominal_value=1  T_nominal_unit=K  Q_specify=off  Q_priority=None  Q=0 J/s  Q_nominal_specify=off  Q_nominal_value=1  Q_nominal_unit=J/s
  WiA-WiB Conduction : fl_lib/Thermal/Thermal Elements/Conductive Heat Transfer  thermal_type=foundation.enum.ConstantVariableTabulated.Constant  wall_geometry=foundation.enum.ConductionWallGeometry.Planar  area=0.002 m^2  thickness=0.1 m  d_in=0.05 m  d_out=0.1 m  L=1 m  th_cond_min=10 W/(K*m)  th_cond=80 W/(m*K)  th_cond_TLU=[413, 401, 392, 383, 371, 357, 342] W/(K*m)  temp_TLU=[200, 273, 400, 600, 800, 1000, 1200] K  T_specify=off  T_priority=None  T=0 K  T_nominal_specify=off  T_nominal_value=1  T_nominal_unit=K  Q_specify=off  Q_priority=None  Q=0 J/s  Q_nominal_specify=off  Q_nominal_value=1  Q_nominal_unit=J/s
  WiA-WiB Convection : fl_lib/Thermal/Thermal Elements/Convective Heat Transfer  thermal_type=foundation.enum.constant_variable.constant  area=0.004 m^2  heat_tr_coeff=200 W/(m^2 * K)  min_heat_tr_coeff=1e-3 W/(K*m^2)  T_specify=off  T_priority=None  T=0 K  T_nominal_specify=off  T_nominal_value=1  T_nominal_unit=K  Q_specify=off  Q_priority=None  Q=0 J/s  Q_nominal_specify=off  Q_nominal_value=1  Q_nominal_unit=J/s
  WiA-WiC Conduction : fl_lib/Thermal/Thermal Elements/Conductive Heat Transfer  thermal_type=foundation.enum.ConstantVariableTabulated.Constant  wall_geometry=foundation.enum.ConductionWallGeometry.Planar  area=0.002 m^2  thickness=0.1 m  d_in=0.05 m  d_out=0.1 m  L=1 m  th_cond_min=10 W/(K*m)  th_cond=80 W/(m*K)  th_cond_TLU=[413, 401, 392, 383, 371, 357, 342] W/(K*m)  temp_TLU=[200, 273, 400, 600, 800, 1000, 1200] K  T_specify=off  T_priority=None  T=0 K  T_nominal_specify=off  T_nominal_value=1  T_nominal_unit=K  Q_specify=off  Q_priority=None  Q=0 J/s  Q_nominal_specify=off  Q_nominal_value=1  Q_nominal_unit=J/s
  WiA-WiC Convection : fl_lib/Thermal/Thermal Elements/Convective Heat Transfer  thermal_type=foundation.enum.constant_variable.constant  area=0.004 m^2  heat_tr_coeff=200 W/(m^2 * K)  min_heat_tr_coeff=1e-3 W/(K*m^2)  T_specify=off  T_priority=None  T=0 K  T_nominal_specify=off  T_nominal_value=1  T_nominal_unit=K  Q_specify=off  Q_priority=None  Q=0 J/s  Q_nominal_specify=off  Q_nominal_value=1  Q_nominal_unit=J/s
  WiB-Amb Convection : fl_lib/Thermal/Thermal Elements/Convective Heat Transfer  thermal_type=foundation.enum.constant_variable.constant  area=0.1 m^2  heat_tr_coeff=20 W/(m^2 * K)  min_heat_tr_coeff=1e-3 W/(K*m^2)  T_specify=off  T_priority=None  T=0 K  T_nominal_specify=off  T_nominal_value=1  T_nominal_unit=K  Q_specify=off  Q_priority=None  Q=0 J/s  Q_nominal_specify=off  Q_nominal_value=1  Q_nominal_unit=J/s
  WiB-Rot Convection : fl_lib/Thermal/Thermal Elements/Convective Heat Transfer  thermal_type=foundation.enum.constant_variable.constant  area=0.02 m^2  heat_tr_coeff=200 W/(m^2 * K)  min_heat_tr_coeff=1e-3 W/(K*m^2)  T_specify=off  T_priority=None  T=0 K  T_nominal_specify=off  T_nominal_value=1  T_nominal_unit=K  Q_specify=off  Q_priority=None  Q=0 J/s  Q_nominal_specify=off  Q_nominal_value=1  Q_nominal_unit=J/s
  WiB-WiC Conduction : fl_lib/Thermal/Thermal Elements/Conductive Heat Transfer  thermal_type=foundation.enum.ConstantVariableTabulated.Constant  wall_geometry=foundation.enum.ConductionWallGeometry.Planar  area=0.002 m^2  thickness=0.1 m  d_in=0.05 m  d_out=0.1 m  L=1 m  th_cond_min=10 W/(K*m)  th_cond=80 W/(m*K)  th_cond_TLU=[413, 401, 392, 383, 371, 357, 342] W/(K*m)  temp_TLU=[200, 273, 400, 600, 800, 1000, 1200] K  T_specify=off  T_priority=None  T=0 K  T_nominal_specify=off  T_nominal_value=1  T_nominal_unit=K  Q_specify=off  Q_priority=None  Q=0 J/s  Q_nominal_specify=off  Q_nominal_value=1  Q_nominal_unit=J/s
  WiB-WiC Convection : fl_lib/Thermal/Thermal Elements/Convective Heat Transfer  thermal_type=foundation.enum.constant_variable.constant  area=0.004 m^2  heat_tr_coeff=200 W/(m^2 * K)  min_heat_tr_coeff=1e-3 W/(K*m^2)  T_specify=off  T_priority=None  T=0 K  T_nominal_specify=off  T_nominal_value=1  T_nominal_unit=K  Q_specify=off  Q_priority=None  Q=0 J/s  Q_nominal_specify=off  Q_nominal_value=1  Q_nominal_unit=J/s
  WiC-Amb Convection : fl_lib/Thermal/Thermal Elements/Convective Heat Transfer  thermal_type=foundation.enum.constant_variable.constant  area=0.1 m^2  heat_tr_coeff=20 W/(m^2 * K)  min_heat_tr_coeff=1e-3 W/(K*m^2)  T_specify=off  T_priority=None  T=0 K  T_nominal_specify=off  T_nominal_value=1  T_nominal_unit=K  Q_specify=off  Q_priority=None  Q=0 J/s  Q_nominal_specify=off  Q_nominal_value=1  Q_nominal_unit=J/s
  WiC-Rot Convection : fl_lib/Thermal/Thermal Elements/Convective Heat Transfer  thermal_type=foundation.enum.constant_variable.constant  area=0.02 m^2  heat_tr_coeff=200 W/(m^2 * K)  min_heat_tr_coeff=1e-3 W/(K*m^2)  T_specify=off  T_priority=None  T=0 K  T_nominal_specify=off  T_nominal_value=1  T_nominal_unit=K  Q_specify=off  Q_priority=None  Q=0 J/s  Q_nominal_specify=off  Q_nominal_value=1  Q_nominal_unit=J/s
  Rotor : PMIOPort  Side=Left
  Winding C : PMIOPort  Port=2  Side=Right
  Winding B : PMIOPort  Port=3  Side=Right
  Winding A : PMIOPort  Port=4  Side=Right
  Env : PMIOPort  Port=5  Side=Left
  connections:
  WiA-Rot Convection/RConn1 -- WiA-WiC Conduction/RConn1 -- WiA-WiC Convection/RConn1 -- WiA-WiB Convection/LConn1 -- WiA-WiB Conduction/LConn1 -- WiA-Amb Convection/LConn1 -- Sensing Temperature WiA/LConn1 -- Winding A/RConn1
  Rotor/RConn1 -- Sensing Temperature Rot/LConn1 -- WiC-Rot Convection/LConn1 -- WiB-Rot Convection/LConn1 -- WiA-Rot Convection/LConn1
  WiA-WiB Convection/RConn1 -- WiA-WiB Conduction/RConn1 -- Sensing Temperature WiB/LConn1 -- WiB-Rot Convection/RConn1 -- Winding B/RConn1 -- WiB-Amb Convection/LConn1 -- WiB-WiC Conduction/LConn1 -- WiB-WiC Convection/LConn1
  WiC-Rot Convection/RConn1 -- Winding C/RConn1 -- WiB-WiC Conduction/RConn1 -- WiB-WiC Convection/RConn1 -- WiC-Amb Convection/LConn1 -- WiA-WiC Convection/LConn1 -- WiA-WiC Conduction/LConn1 -- Sensing Temperature WiC/LConn1
  WiA-Amb Convection/RConn1 -- Env/RConn1 -- WiC-Amb Convection/RConn1 -- WiB-Amb Convection/RConn1
